simulink model "SCDalgo_confstate_harness"  (R2019a)
settings: Solver=FixedStepAuto  StartTime=0.0  StopTime=2.5  FixedStep=1e-4  RelTol=1e-3
undefined symbols (not defined in the file or in its folder): SCDalgo_confstate_fp
settings Model: DataDictionary=SCDalgo_confstate.sldd  Creator=ffelici  LastModifiedBy=marceca

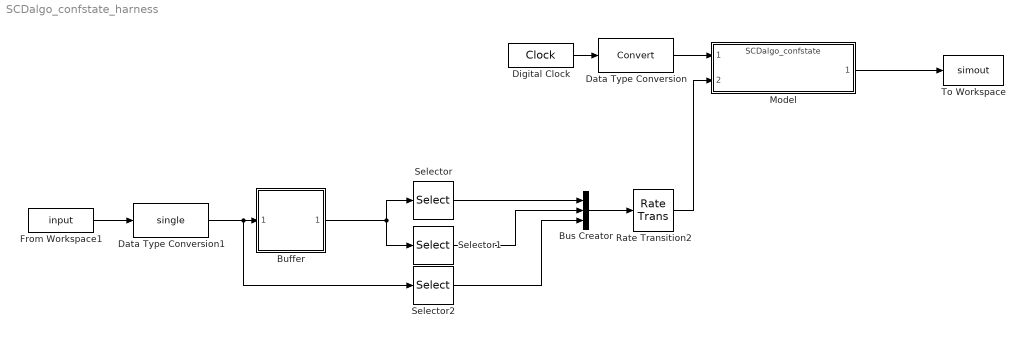
== system SCDalgo_confstate_harness ==
  Buffer : Subsystem
  Bus Creator : BusCreator  Inputs=3  OutDataTypeStr=Bus: SCDconfstate_in
      settings: InheritFromInputs=off
  Data Type Conversion : DataTypeConversion
  Data Type Conversion1 : DataTypeConversion  OutDataTypeStr=single
  Digital Clock : DigitalClock  SampleTime=1e-4
  From Workspace1 : FromWorkspace  VariableName=input  SampleTime=0
  Model : ModelReference  ModelNameDialog=SCDalgo_confstate.slx  SimulationMode=Normal  ModelReferenceVersion=1.745  SimulationMode=Normal
  Rate Transition2 : RateTransition  OutPortSampleTime=1e-3
  Selector : Selector  NumberOfDimensions=2  InputPortWidth=3  IndexOptions=Select all,Index vector (dialog)  Indices=[1 3],1  OutputSizes=1,1
  Selector1 : Selector  NumberOfDimensions=2  InputPortWidth=3  IndexOptions=Select all,Index vector (dialog)  Indices=[1 3],2  OutputSizes=1,1
  Selector2 : Selector  IndexOptions=Index vector (dialog)  Indices=3  OutputSizes=1
  To Workspace : ToWorkspace  VariableName=simout  SaveFormat=Timeseries  SampleTime=-1
  wires:
  Model/1 -> To Workspace/1
  Digital Clock/1 -> Data Type Conversion/1
  Data Type Conversion/1 -> Model/1
  From Workspace1/1 -> Data Type Conversion1/1
  Buffer/1(window_t_10khz) -> Selector1/1, Selector/1
  Selector/1 -> Bus Creator/1
  Selector1/1 -> Bus Creator/2
  Bus Creator/1 -> Rate Transition2/1
  Rate Transition2/1 -> Model/2
  Selector2/1 -> Bus Creator/3
  Data Type Conversion1/1 -> Selector2/1, Buffer/1(data_i_10khz)

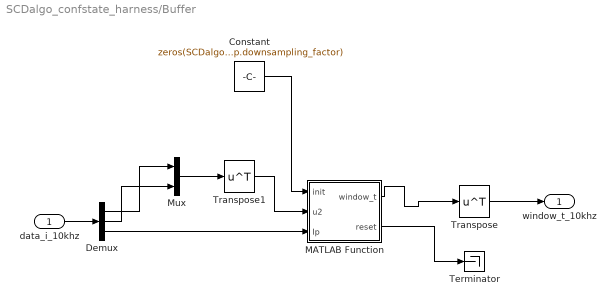
== system SCDalgo_confstate_harness/Buffer ==
  data_i_10khz : Inport
  Constant : Constant  Value=zeros(SCDalgo_confstate_fp.n_signals, SCDalgo_confstate_fp.downsampling_factor)
  Demux : Demux  Outputs=3
  MATLAB Function : MATLAB Function  TreatAsAtomicUnit=on
  Mux : Mux  Inputs=2
  Terminator : Terminator
  Transpose : Math  Operator=transpose  SaturateOnIntegerOverflow=on
  Transpose1 : Math  Operator=transpose  SaturateOnIntegerOverflow=on
  window_t_10khz : Outport
  wires:
  MATLAB Function/1(window_t) -> Transpose/1
  Transpose/1 -> window_t_10khz/1
  data_i_10khz/1 -> Demux/1
  Demux/3 -> MATLAB Function/3(Ip)
  Demux/1 -> Mux/1
  Demux/2 -> Mux/2
  Mux/1 -> Transpose1/1
  Transpose1/1 -> MATLAB Function/2(u2)
  MATLAB Function/2(reset) -> Terminator/1
  Constant/1 -> MATLAB Function/1(init)

== matlab function SCDalgo_confstate_harness/Buffer/MATLAB Function ==
  data: init input; u2 input; window_t output single; Ip input; reset output; SCDalgo_confstate_tp parameter
function [window_t, reset]  = buffer(init, u2, Ip, SCDalgo_confstate_tp)
%#codegen
[window_t, reset] =buffer_func(init, u2, Ip, SCDalgo_confstate_tp);
